simulink library "Environment_lib"  (R2018b)
settings: Solver=VariableStepAuto  StartTime=0.0  StopTime=10.0  RelTol=1e-3
undefined symbols (not defined in the file): B_eci_T, dist_torque_Nm, eclipse, env_acc_mps2, fswParams, sc2sun_eci_unit, simParams
libraries: vrlib x1, gravityGrad_Lib x1, atmoDrag_lib x1, magField_lib x1, solarPressure_lib x1, clock_lib x1, orbit_data_bus x1, time_Lib x1
settings Model: Creator=Taylor  LastModifiedBy=taylorreynolds

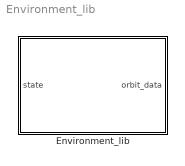
== system Environment_lib ==
  Environment_lib : Subsystem

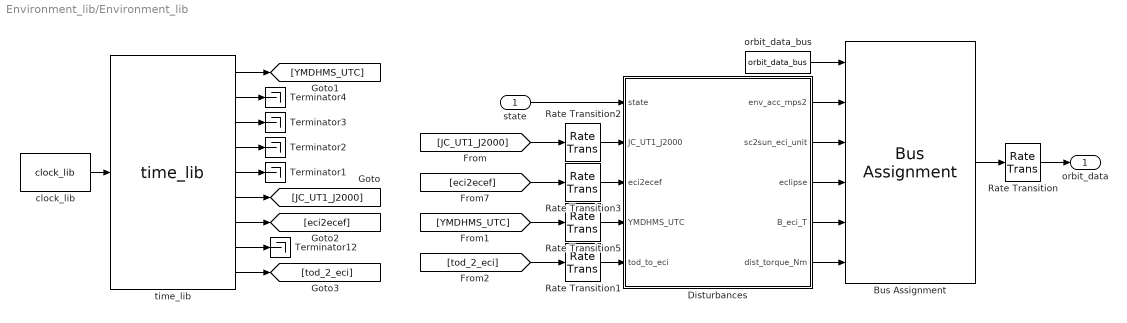
== system Environment_lib/Environment_lib ==
  state : Inport  OutDataTypeStr=Bus: state
  Bus Assignment : BusAssignment  AssignedSignals=env_acc_mps2,sc2sun_eci_unit,eclipse,B_eci_T,dist_torque_Nm
  Disturbances : Subsystem
  Rate Transition{,1..3,5} (5 alike) : RateTransition  OutPortSampleTime=simParams.sample_time_s
  Terminator{1..4,12} (5 alike) : Terminator
  clock_lib : clock_lib/clock_lib  SystemSampleTime=-1
  orbit_data_bus : orbit_data_bus/orbit_data_bus  SystemSampleTime=-1
  "time_lib " : time_Lib/time_lib    SystemSampleTime=-1
  orbit_data : Outport  OutDataTypeStr=Bus: orbit_data
  wires:
  Rate Transition3/1 -> Disturbances/3(eci2ecef)
  Rate Transition5/1 -> Disturbances/4(YMDHMS_UTC)
  Rate Transition2/1 -> Disturbances/2(JC_UT1_J2000)
  [JC_UT1_J2000] -> Rate Transition2/1
  [eci2ecef] -> Rate Transition3/1
  clock_lib/1 -> "time_lib "/1
  [YMDHMS_UTC] -> Rate Transition5/1
  Disturbances/1(env_acc_mps2) -> Bus Assignment/2
  state/1 -> Disturbances/1(state)
  orbit_data_bus/1 -> Bus Assignment/1
  Bus Assignment/1 -> Rate Transition/1
  "time_lib "/8 -> Terminator12/1
  Rate Transition/1 -> orbit_data/1
  "time_lib "/1 -> [YMDHMS_UTC]
  "time_lib "/6 -> [JC_UT1_J2000]
  "time_lib "/7 -> [eci2ecef]
  "time_lib "/5 -> Terminator1/1
  "time_lib "/4 -> Terminator2/1
  "time_lib "/3 -> Terminator3/1
  "time_lib "/2 -> Terminator4/1
  Disturbances/2(sc2sun_eci_unit) -> Bus Assignment/3
  Disturbances/3(eclipse) -> Bus Assignment/4
  Disturbances/4(B_eci_T) -> Bus Assignment/5
  Disturbances/5(dist_torque_Nm) -> Bus Assignment/6
  "time_lib "/9 -> [tod_2_eci]
  Rate Transition1/1 -> Disturbances/5(tod_to_eci)
  [tod_2_eci] -> Rate Transition1/1

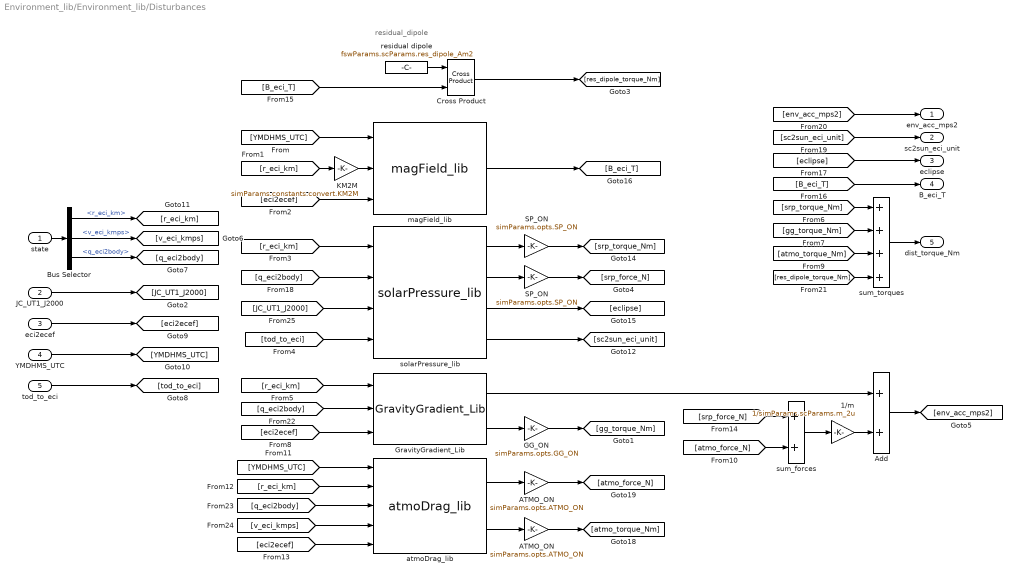
== system Environment_lib/Environment_lib/Disturbances ==
  note: residual_dipole
  state : Inport  OutDataTypeStr=Bus: state
  JC_UT1_J2000 : Inport  Port=2
  eci2ecef : Inport  Port=3
  YMDHMS_UTC : Inport  Port=4
  tod_to_eci : Inport  Port=5
  1/m : Gain  Gain=1/simParams.scParams.m_2u
  ATMO_ON : Gain  Gain=simParams.opts.ATMO_ON
  "ATMO_ON " : Gain  Gain=simParams.opts.ATMO_ON
  Add : Sum
  Bus Selector : BusSelector  OutputSignals=r_eci_km,v_eci_kmps,q_eci2body
  Cross Product : vrlib/Utilities/Cross Product
      settings: SourceProductBaseCode=VR
  GG_ON : Gain  Gain=simParams.opts.GG_ON
  "GravityGradient_Lib " : gravityGrad_Lib/GravityGradient_Lib   SystemSampleTime=-1
  KM2M : Gain  Gain=simParams.constants.convert.KM2M
  SP_ON : Gain  Gain=simParams.opts.SP_ON
  "SP_ON " : Gain  Gain=simParams.opts.SP_ON
  atmoDrag_lib : atmoDrag_lib/atmoDrag_lib  SystemSampleTime=-1
  magField_lib : magField_lib/magField_lib  SystemSampleTime=-1
  residual dipole : Constant  Value=fswParams.scParams.res_dipole_Am2
  solarPressure_lib : solarPressure_lib/solarPressure_lib  SystemSampleTime=-1
  sum_forces : Sum
  sum_torques : Sum  Inputs=++++
  env_acc_mps2 : Outport
  sc2sun_eci_unit : Outport  Port=2
  eclipse : Outport  Port=3
  B_eci_T : Outport  Port=4
  dist_torque_Nm : Outport  Port=5
  wires:
  solarPressure_lib/3 -> [eclipse]
  JC_UT1_J2000/1 -> [JC_UT1_J2000]
  sum_forces/1 -> 1/m/1
  Add/1 -> [env_acc_mps2]
  1/m/1 -> Add/2
  atmoDrag_lib/2 -> "ATMO_ON "/1
  atmoDrag_lib/1 -> ATMO_ON/1
  "ATMO_ON "/1 -> [atmo_torque_Nm]
  state/1 -> Bus Selector/1
  [r_eci_km] -> solarPressure_lib/1
  eci2ecef/1 -> [eci2ecef]
  [eci2ecef] -> atmoDrag_lib/5
  [YMDHMS_UTC] -> atmoDrag_lib/1
  "SP_ON "/1 -> [srp_torque_Nm]
  [srp_torque_Nm] -> sum_torques/1
  GG_ON/1 -> [gg_torque_Nm]
  [gg_torque_Nm] -> sum_torques/2
  [eci2ecef] -> "GravityGradient_Lib "/3
  sum_torques/1 -> dist_torque_Nm/1
  [atmo_torque_Nm] -> sum_torques/3
  [atmo_force_N] -> sum_forces/2
  [srp_force_N] -> sum_forces/1
  ATMO_ON/1 -> [atmo_force_N]
  SP_ON/1 -> [srp_force_N]
  "GravityGradient_Lib "/1 -> Add/1
  "GravityGradient_Lib "/2 -> GG_ON/1
  KM2M/1 -> magField_lib/2
  YMDHMS_UTC/1 -> [YMDHMS_UTC]
  [YMDHMS_UTC] -> magField_lib/1
  [eci2ecef] -> magField_lib/3
  magField_lib/1 -> [B_eci_T]
  solarPressure_lib/4 -> [sc2sun_eci_unit]
  [JC_UT1_J2000] -> solarPressure_lib/3
  [B_eci_T] -> B_eci_T/1
  solarPressure_lib/2 -> SP_ON/1
  solarPressure_lib/1 -> "SP_ON "/1
  [eclipse] -> eclipse/1
  [sc2sun_eci_unit] -> sc2sun_eci_unit/1
  [env_acc_mps2] -> env_acc_mps2/1
  [res_dipole_torque_Nm] -> sum_torques/4
  Cross Product/1 -> [res_dipole_torque_Nm]
  residual dipole/1 -> Cross Product/1
  [B_eci_T] -> Cross Product/2
  Bus Selector/1 -> [r_eci_km]  "<r_eci_km>"
  [r_eci_km] -> KM2M/1
  Bus Selector/3 -> [q_eci2body]  "<q_eci2body>"
  Bus Selector/2 -> [v_eci_kmps]  "<v_eci_kmps>"
  [q_eci2body] -> solarPressure_lib/2
  [r_eci_km] -> "GravityGradient_Lib "/1
  [q_eci2body] -> "GravityGradient_Lib "/2
  [r_eci_km] -> atmoDrag_lib/2
  [q_eci2body] -> atmoDrag_lib/3
  [v_eci_kmps] -> atmoDrag_lib/4
  tod_to_eci/1 -> [tod_to_eci]
  [tod_to_eci] -> solarPressure_lib/4
